simulink subsystem "non_linear_plant"  (R2022b)
settings: Solver=VariableStepAuto  StartTime=0.0  StopTime=10.0  RelTol=1e-3
undefined symbols (not defined in the file or in its folder): param
libraries: simulink x1
settings Model: Creator=Alex Zhen  LastModifiedBy=Alex Zhen

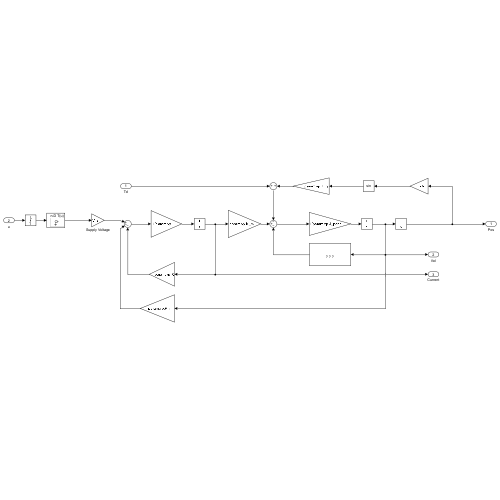
[thumbnail: Simulink's stored preview of the top-level diagram]
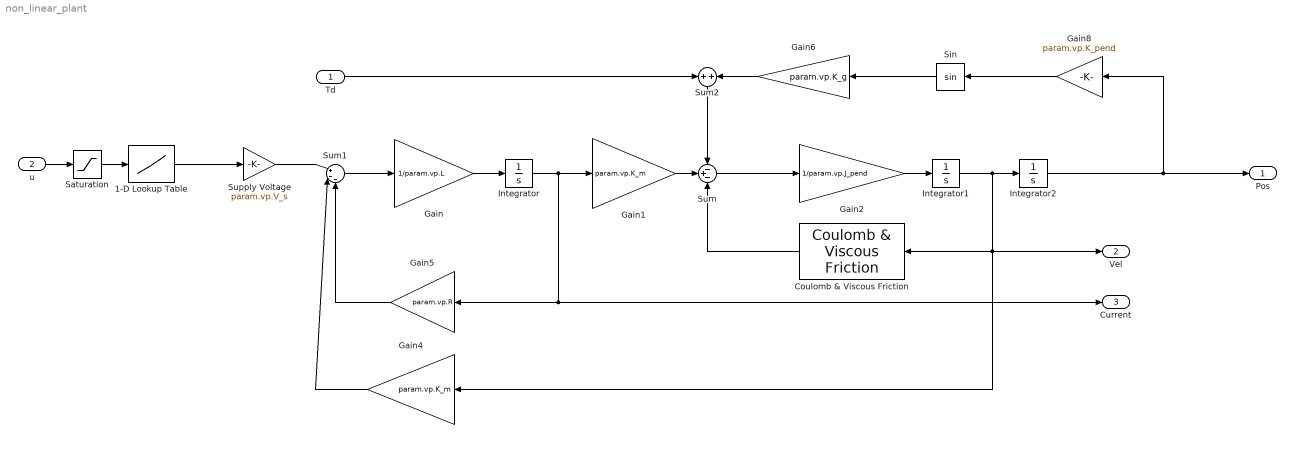
== system non_linear_plant ==
  Td : Inport
  u : Inport  Port=2
  1-D Lookup Table : Lookup_n-D  NumberOfTableDimensions=1  BreakpointsForDimension1=[-1,-0.96,-0.1,-0.06,-0.04,0,0.04,0.06,0.1,0.96,1]  Table=[-10.8,-10.8,-2,-1,-0,0,0,1,2,10.8,10.8]/param.vp.V_s  InternalRulePriority=Speed  RndMeth=Simplest
  Coulomb & Viscous Friction : simulink/Discontinuities/Coulomb & Viscous Friction  offset=param.vp.Friction_static  gain=param.vp.b
  Gain : Gain  Gain=1/param.vp.L
  Gain1 : Gain  Gain=param.vp.K_m
  Gain2 : Gain  Gain=1/param.vp.J_pend
  Gain4 : Gain  Gain=param.vp.K_m
  Gain5 : Gain  Gain=param.vp.R
  Gain6 : Gain  Gain=param.vp.K_g
  Gain8 : Gain  Gain=param.vp.K_pend
  Integrator : Integrator
  Integrator1 : Integrator
  Integrator2 : Integrator
  Saturation : Saturate  UpperLimit=param.vp.saturation  LowerLimit=-param.vp.saturation
  Sin : Trigonometry
  Sum : Sum  Inputs=-+-
  Sum1 : Sum  Inputs=|+--
  Sum2 : Sum
  Supply Voltage : Gain  Gain=param.vp.V_s
  Pos : Outport
  Vel : Outport  Port=2
  Current : Outport  Port=3
  wires:
  Sin/1 -> Gain6/1
  Gain8/1 -> Sin/1
  Sum/1 -> Gain2/1
  Gain4/1 -> Sum1/2
  Sum2/1 -> Sum/1
  Gain2/1 -> Integrator1/1
  Integrator1/1 -> Coulomb & Viscous Friction/1, Vel/1, Gain4/1, Integrator2/1
  Gain/1 -> Integrator/1
  Integrator/1 -> Gain1/1, Current/1, Gain5/1
  Gain5/1 -> Sum1/3
  Gain6/1 -> Sum2/2
  Integrator2/1 -> Pos/1, Gain8/1
  Sum1/1 -> Gain/1
  Td/1 -> Sum2/1
  Coulomb & Viscous Friction/1 -> Sum/3
  Gain1/1 -> Sum/2
  1-D Lookup Table/1 -> Supply Voltage/1
  u/1 -> Saturation/1
  Saturation/1 -> 1-D Lookup Table/1
  Supply Voltage/1 -> Sum1/1
